simulink model "inverter_spwm_sixty_phases"  (R2024b)
settings: Solver=VariableStepAuto  StartTime=0.0  StopTime=0.1  RelTol=1e-3
libraries: spsMosfetLib x132, spsSeriesRLCBranchLib x65, spsCurrentMeasurementLib x64, spsVoltageMeasurementLib x64, spsTriangleGeneratorLib x20, spsDCVoltageSourceLib x4, spsGroundLib x2, spsThreePhaseSeriesRLCBranchLib x1, sps_lib x1
(part 2 of 2)

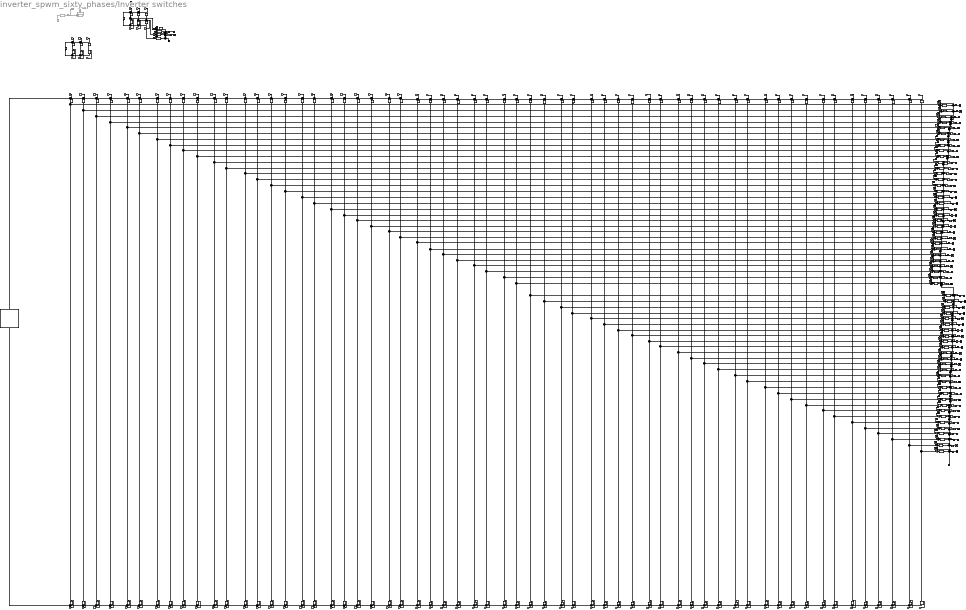
== system inverter_spwm_sixty_phases/Inverter switches ==
  Current Measurement : spsCurrentMeasurementLib/Current Measurement  Commented=on  PhasorSimulation=off  OutputType=Complex  PSBequivalent=0
  Current Measurement{1..47,49..52,55..66} (63 alike) : spsCurrentMeasurementLib/Current Measurement  PhasorSimulation=off  OutputType=Complex  PSBequivalent=0
  DC Voltage Source : spsDCVoltageSourceLib/DC Voltage Source  Amplitude=48  Measurements=None
  DC Voltage Source1 : spsDCVoltageSourceLib/DC Voltage Source  Commented=on  Amplitude=48  Measurements=None
  DC Voltage Source2 : spsDCVoltageSourceLib/DC Voltage Source  Amplitude=48  Measurements=None
  DC Voltage Source3 : spsDCVoltageSourceLib/DC Voltage Source  Amplitude=48  Measurements=None
  Ground : spsGroundLib/Ground  LConnTagsString=a
  Ground1 : spsGroundLib/Ground  LConnTagsString=a
  Mosfet{1..5,7..11,13..132} (130 alike) : spsMosfetLib/Mosfet  Ron=ron  Lon=0  Rd=rd  Vfd=fv  IC=0  Rs=0  Cs=0  Measurements=on
  Mosfet12 : spsMosfetLib/Mosfet  Ron=ron  Lon=0  Rd=rd  Vfd=fv  IC=0  Rs=0  Cs=0  Measurements=off
  Mosfet6 : spsMosfetLib/Mosfet  Ron=ron  Lon=0  Rd=rd  Vfd=fv  IC=0  Rs=0  Cs=0  Measurements=off
  Scope{,1,3..4,6..118,127..134} (125 alike) : Scope
  Scope2 : Scope  Commented=on
  Scope5 : Scope  Commented=on
  Series RLC Branch : spsSeriesRLCBranchLib/Series RLC Branch  Commented=on  LConnTagsString=__new0  RConnTagsString=__new0  BranchType=RC  Resistance=0.005  Inductance=0  SetiL0=off  InitialCurrent=0  Capacitance=0.02  Setx0=off  InitialVoltage=0  Measurements=None
  Series RLC Branch1 : spsSeriesRLCBranchLib/Series RLC Branch  Commented=on  LConnTagsString=__new0  RConnTagsString=__new0  BranchType=R  Resistance=0.0005  Inductance=1e-3  SetiL0=off  InitialCurrent=0  Capacitance=1e-6  Setx0=off  InitialVoltage=0  Measurements=None
  Series RLC Branch{2..50,54..57,59..68} (63 alike) : spsSeriesRLCBranchLib/Series RLC Branch  LConnTagsString=__new0  RConnTagsString=__new0  BranchType=RL  Resistance=1.0274  Inductance=0.0027  SetiL0=off  InitialCurrent=0  Capacitance=1e-6  Setx0=off  InitialVoltage=0  Measurements=None
  Three-Phase Series RLC Branch1 : spsThreePhaseSeriesRLCBranchLib/Three-Phase Series RLC Branch  LConnTagsString=A|B|C  RConnTagsString=A|B|C  BranchType=RL  Resistance=1.0274  Inductance=0.0027  Capacitance=1e-6  Measurements=Branch voltages
  Voltage Measurement : spsVoltageMeasurementLib/Voltage Measurement  Commented=on  PhasorSimulation=off  OutputType=Complex  PSBequivalent=0
  Voltage Measurement{1..47,50..53,56..67} (63 alike) : spsVoltageMeasurementLib/Voltage Measurement  PhasorSimulation=off  OutputType=Complex  PSBequivalent=0
  wires:
  [s6] -> Mosfet6/1
  [s1] -> Mosfet1/1
  [s3] -> Mosfet2/1
  [s5] -> Mosfet3/1
  [s2] -> Mosfet4/1
  [s4] -> Mosfet5/1
  Voltage Measurement/1 -> Scope5/1
  Current Measurement/1 -> Scope2/1
  Current Measurement1/1 -> Scope6/1
  Voltage Measurement2/1 -> Scope7/1
  Voltage Measurement3/1 -> Scope/1
  Current Measurement2/1 -> Scope1/1
  Current Measurement3/1 -> Scope3/1
  [s1] -> Mosfet7/1
  [s4] -> Mosfet11/1
  [s6] -> Mosfet12/1
  [s2] -> Mosfet10/1
  [s5] -> Mosfet9/1
  [s3] -> Mosfet8/1
  [s1] -> Mosfet13/1
  [s3] -> Mosfet14/1
  [s5] -> Mosfet17/1
  [s7] -> Mosfet19/1
  [s9] -> Mosfet21/1
  [s11] -> Mosfet23/1
  [s2] -> Mosfet15/1
  [s4] -> Mosfet16/1
  [s6] -> Mosfet18/1
  [s8] -> Mosfet20/1
  [s10] -> Mosfet22/1
  [s12] -> Mosfet24/1
  [s24] -> Mosfet36/1
  [s18] -> Mosfet30/1
  [s16] -> Mosfet28/1
  [s14] -> Mosfet27/1
  [s20] -> Mosfet32/1
  [s23] -> Mosfet35/1
  [s21] -> Mosfet33/1
  [s22] -> Mosfet34/1
  [s19] -> Mosfet31/1
  [s17] -> Mosfet29/1
  [s15] -> Mosfet26/1
  [s13] -> Mosfet25/1
  [s36] -> Mosfet48/1
  [s30] -> Mosfet42/1
  [s28] -> Mosfet40/1
  [s26] -> Mosfet39/1
  [s32] -> Mosfet44/1
  [s35] -> Mosfet47/1
  [s33] -> Mosfet45/1
  [s45] -> Mosfet57/1
  [s47] -> Mosfet59/1
  [s44] -> Mosfet56/1
  [s46] -> Mosfet58/1
  [s34] -> Mosfet46/1
  [s38] -> Mosfet51/1
  [s42] -> Mosfet54/1
  [s48] -> Mosfet60/1
  [s43] -> Mosfet55/1
  [s37] -> Mosfet49/1
  [s39] -> Mosfet50/1
  [s29] -> Mosfet41/1
  [s40] -> Mosfet52/1
  [s31] -> Mosfet43/1
  [s41] -> Mosfet53/1
  [s25] -> Mosfet37/1
  [s27] -> Mosfet38/1
  [s108] -> Mosfet72/1
  [s102] -> Mosfet66/1
  [s100] -> Mosfet64/1
  [s98] -> Mosfet63/1
  [s104] -> Mosfet68/1
  [s107] -> Mosfet71/1
  [s105] -> Mosfet69/1
  [s117] -> Mosfet81/1
  [s119] -> Mosfet83/1
  [s116] -> Mosfet80/1
  [s118] -> Mosfet82/1
  [s106] -> Mosfet70/1
  [s110] -> Mosfet75/1
  [s114] -> Mosfet78/1
  [s120] -> Mosfet84/1
  [s115] -> Mosfet79/1
  [s109] -> Mosfet73/1
  [s111] -> Mosfet74/1
  [s101] -> Mosfet65/1
  [s112] -> Mosfet76/1
  [s103] -> Mosfet67/1
  [s113] -> Mosfet77/1
  [s97] -> Mosfet61/1
  [s99] -> Mosfet62/1
  [s60] -> Mosfet96/1
  [s54] -> Mosfet90/1
  [s88] -> Mosfet124/1
  [s77] -> Mosfet113/1
  [s75] -> Mosfet110/1
  [s89] -> Mosfet125/1
  [s73] -> Mosfet109/1
  [s93] -> Mosfet129/1
  [s87] -> Mosfet122/1
  [s95] -> Mosfet131/1
  [s94] -> Mosfet130/1
  [s96] -> Mosfet132/1
  [s90] -> Mosfet126/1
  [s86] -> Mosfet123/1
  [s81] -> Mosfet117/1
  [s82] -> Mosfet118/1
  [s92] -> Mosfet128/1
  [s91] -> Mosfet127/1
  [s83] -> Mosfet119/1
  [s74] -> Mosfet111/1
  [s76] -> Mosfet112/1
  [s80] -> Mosfet116/1
  [s79] -> Mosfet115/1
  [s52] -> Mosfet88/1
  [s50] -> Mosfet87/1
  [s84] -> Mosfet120/1
  [s56] -> Mosfet92/1
  [s59] -> Mosfet95/1
  [s57] -> Mosfet93/1
  [s69] -> Mosfet105/1
  [s71] -> Mosfet107/1
  [s68] -> Mosfet104/1
  [s70] -> Mosfet106/1
  [s78] -> Mosfet114/1
  [s58] -> Mosfet94/1
  [s62] -> Mosfet99/1
  [s66] -> Mosfet102/1
  [s72] -> Mosfet108/1
  [s67] -> Mosfet103/1
  [s61] -> Mosfet97/1
  [s63] -> Mosfet98/1
  [s53] -> Mosfet89/1
  [s64] -> Mosfet100/1
  [s55] -> Mosfet91/1
  [s65] -> Mosfet101/1
  [s49] -> Mosfet85/1
  [s51] -> Mosfet86/1
  [s85] -> Mosfet121/1
  Current Measurement5/1 -> Scope10/1
  Voltage Measurement5/1 -> Scope9/1
  Voltage Measurement4/1 -> Scope8/1
  Current Measurement4/1 -> Scope4/1
  Current Measurement6/1 -> Scope12/1
  Voltage Measurement6/1 -> Scope13/1
  Voltage Measurement7/1 -> Scope14/1
  Current Measurement7/1 -> Scope11/1
  Current Measurement11/1 -> Scope16/1
  Voltage Measurement11/1 -> Scope19/1
  Voltage Measurement10/1 -> Scope18/1
  Current Measurement10/1 -> Scope17/1
  Current Measurement8/1 -> Scope20/1
  Voltage Measurement8/1 -> Scope21/1
  Voltage Measurement9/1 -> Scope22/1
  Current Measurement9/1 -> Scope15/1
  Current Measurement19/1 -> Scope28/1
  Voltage Measurement19/1 -> Scope35/1
  Voltage Measurement18/1 -> Scope34/1
  Current Measurement18/1 -> Scope33/1
  Current Measurement12/1 -> Scope30/1
  Voltage Measurement12/1 -> Scope31/1
  Voltage Measurement13/1 -> Scope32/1
  Current Measurement13/1 -> Scope29/1
  Current Measurement17/1 -> Scope24/1
  Voltage Measurement17/1 -> Scope27/1
  Voltage Measurement16/1 -> Scope26/1
  Current Measurement16/1 -> Scope25/1
  Current Measurement14/1 -> Scope36/1
  Voltage Measurement14/1 -> Scope37/1
  Voltage Measurement15/1 -> Scope38/1
  Current Measurement15/1 -> Scope23/1
  Current Measurement25/1 -> Scope52/1
  Voltage Measurement25/1 -> Scope67/1
  Voltage Measurement24/1 -> Scope66/1
  Current Measurement24/1 -> Scope65/1
  Current Measurement26/1 -> Scope54/1
  Voltage Measurement26/1 -> Scope55/1
  Voltage Measurement27/1 -> Scope56/1
  Current Measurement27/1 -> Scope53/1
  Current Measurement23/1 -> Scope58/1
  Voltage Measurement23/1 -> Scope61/1
  Voltage Measurement22/1 -> Scope60/1
  Current Measurement22/1 -> Scope59/1
  Current Measurement28/1 -> Scope62/1
  Voltage Measurement28/1 -> Scope63/1
  Voltage Measurement29/1 -> Scope64/1
  Current Measurement29/1 -> Scope57/1
  Current Measurement35/1 -> Scope44/1
  Voltage Measurement35/1 -> Scope51/1
  Voltage Measurement34/1 -> Scope50/1
  Current Measurement34/1 -> Scope49/1
  Current Measurement20/1 -> Scope46/1
  Voltage Measurement20/1 -> Scope47/1
  Voltage Measurement21/1 -> Scope48/1
  Current Measurement21/1 -> Scope45/1
  Current Measurement33/1 -> Scope40/1
  Voltage Measurement33/1 -> Scope43/1
  Voltage Measurement32/1 -> Scope42/1
  Current Measurement32/1 -> Scope41/1
  Current Measurement30/1 -> Scope68/1
  Voltage Measurement30/1 -> Scope69/1
  Voltage Measurement31/1 -> Scope70/1
  Current Measurement31/1 -> Scope39/1
  Current Measurement56/1 -> Scope100/1
  Voltage Measurement57/1 -> Scope132/1
  Voltage Measurement56/1 -> Scope131/1
  Current Measurement55/1 -> Scope130/1
  Current Measurement57/1 -> Scope103/1
  Voltage Measurement58/1 -> Scope104/1
  Voltage Measurement59/1 -> Scope105/1
  Current Measurement58/1 -> Scope102/1
  Current Measurement47/1 -> Scope107/1
  Voltage Measurement47/1 -> Scope110/1
  Voltage Measurement46/1 -> Scope109/1
  Current Measurement46/1 -> Scope108/1
  Current Measurement59/1 -> Scope111/1
  Voltage Measurement60/1 -> Scope112/1
  Voltage Measurement61/1 -> Scope113/1
  Current Measurement60/1 -> Scope106/1
  Current Measurement52/1 -> Scope115/1
  Voltage Measurement53/1 -> Scope118/1
  Voltage Measurement52/1 -> Scope117/1
  Current Measurement51/1 -> Scope116/1
  Current Measurement49/1 -> Scope127/1
  Voltage Measurement50/1 -> Scope128/1
  Voltage Measurement51/1 -> Scope129/1
  Current Measurement50/1 -> Scope114/1
  Current Measurement41/1 -> Scope84/1
  Voltage Measurement41/1 -> Scope99/1
  Voltage Measurement40/1 -> Scope98/1
  Current Measurement40/1 -> Scope97/1
  Current Measurement42/1 -> Scope86/1
  Voltage Measurement42/1 -> Scope87/1
  Voltage Measurement43/1 -> Scope88/1
  Current Measurement43/1 -> Scope85/1
  Current Measurement39/1 -> Scope90/1
  Voltage Measurement39/1 -> Scope93/1
  Voltage Measurement38/1 -> Scope92/1
  Current Measurement38/1 -> Scope91/1
  Current Measurement44/1 -> Scope94/1
  Voltage Measurement44/1 -> Scope95/1
  Voltage Measurement45/1 -> Scope96/1
  Current Measurement45/1 -> Scope89/1
  Current Measurement66/1 -> Scope76/1
  Voltage Measurement67/1 -> Scope83/1
  Voltage Measurement66/1 -> Scope82/1
  Current Measurement65/1 -> Scope81/1
  Current Measurement36/1 -> Scope78/1
  Voltage Measurement36/1 -> Scope79/1
  Voltage Measurement37/1 -> Scope80/1
  Current Measurement37/1 -> Scope77/1
  Current Measurement64/1 -> Scope72/1
  Voltage Measurement65/1 -> Scope75/1
  Voltage Measurement64/1 -> Scope74/1
  Current Measurement63/1 -> Scope73/1
  Current Measurement61/1 -> Scope101/1
  Voltage Measurement62/1 -> Scope133/1
  Voltage Measurement63/1 -> Scope134/1
  Current Measurement62/1 -> Scope71/1
  connections:
  Mosfet2/LConn1 -- DC Voltage Source/RConn1 -- Mosfet1/LConn1 -- Mosfet3/LConn1
  Mosfet3/RConn1 -- Current Measurement3/LConn1 -- Mosfet6/LConn1
  Mosfet2/RConn1 -- Current Measurement2/LConn1 -- Mosfet5/LConn1
  Mosfet1/RConn1 -- Current Measurement1/LConn1 -- Mosfet4/LConn1
  Mosfet5/RConn1 -- Mosfet4/RConn1 -- DC Voltage Source/LConn1 -- Mosfet6/RConn1
  Current Measurement/RConn1 -- Voltage Measurement/LConn1 -- Series RLC Branch/LConn1
  Voltage Measurement/LConn2 -- Series RLC Branch/RConn1
  Series RLC Branch1/RConn1 -- Current Measurement/LConn1
  DC Voltage Source1/RConn1 -- Series RLC Branch1/LConn1
  Current Measurement1/RConn1 -- Voltage Measurement2/LConn1 -- Series RLC Branch2/LConn1
  Voltage Measurement2/LConn2 -- Series RLC Branch4/RConn1 -- Ground/LConn1 -- Voltage Measurement3/LConn2 -- Series RLC Branch3/RConn1 -- Series RLC Branch2/RConn1
  Series RLC Branch3/LConn1 -- Voltage Measurement3/LConn1 -- Current Measurement2/RConn1
  Series RLC Branch4/LConn1 -- Current Measurement3/RConn1
  Mosfet12/LConn1 -- Mosfet9/RConn1
  DC Voltage Source2/LConn1 -- Mosfet11/RConn1 -- Mosfet12/RConn1 -- Mosfet10/RConn1
  Mosfet9/LConn1 -- Mosfet8/LConn1 -- DC Voltage Source2/RConn1 -- Mosfet7/LConn1
  Mosfet11/LConn1 -- Mosfet8/RConn1
  Mosfet7/RConn1 -- Mosfet10/LConn1
  Mosfet15/LConn1 -- Current Measurement5/LConn1 -- Mosfet13/RConn1
  Mosfet16/LConn1 -- Mosfet14/RConn1 -- Current Measurement4/LConn1
  Mosfet18/LConn1 -- Mosfet17/RConn1 -- Current Measurement7/LConn1
  Current Measurement55/LConn1 -- Mosfet64/LConn1 -- Mosfet62/RConn1
  Current Measurement60/LConn1 -- Mosfet70/LConn1 -- Mosfet69/RConn1
  Current Measurement38/LConn1 -- Mosfet132/LConn1 -- Mosfet131/RConn1
  Mosfet80/LConn1 -- Current Measurement49/LConn1 -- Mosfet79/RConn1
  Mosfet82/LConn1 -- Mosfet81/RConn1 -- Current Measurement52/LConn1
  Mosfet84/LConn1 -- Mosfet83/RConn1 -- Current Measurement51/LConn1
  Current Measurement57/LConn1 -- Mosfet68/LConn1 -- Mosfet67/RConn1
  Current Measurement46/LConn1 -- Mosfet76/LConn1 -- Mosfet74/RConn1
  Mosfet81/LConn1 -- Mosfet83/LConn1 -- Mosfet79/LConn1 -- Mosfet77/LConn1 -- Mosfet73/LConn1 -- Mosfet61/LConn1 -- Mosfet129/LConn1 -- Mosfet127/LConn1 -- Mosfet125/LConn1 -- Mosfet122/LConn1 -- Mosfet121/LConn1 -- Mosfet119/LConn1 -- Mosfet117/LConn1 -- Mosfet97/LConn1 -- Mosfet85/LConn1 -- Mosfet49/LConn1 -- Mosfet25/LConn1 -- DC Voltage Source3/RConn1 -- Mosfet13/LConn1 -- Mosfet14/LConn1 -- Mosfet17/LConn1 -- Mosfet19/LConn1 -- Mosfet21/LConn1 -- Mosfet23/LConn1 -- Mosfet26/LConn1 -- Mosfet29/LConn1 -- Mosfet31/LConn1 -- Mosfet33/LConn1 -- Mosfet35/LConn1 -- Mosfet37/LConn1 -- Mosfet38/LConn1 -- Mosfet41/LConn1 -- Mosfet43/LConn1 -- Mosfet45/LConn1 -- Mosfet47/LConn1 -- Mosfet50/LConn1 -- Mosfet53/LConn1 -- Mosfet55/LConn1 -- Mosfet57/LConn1 -- Mosfet59/LConn1 -- Mosfet86/LConn1 -- Mosfet89/LConn1 -- Mosfet91/LConn1 -- Mosfet93/LConn1 -- Mosfet95/LConn1 -- Mosfet98/LConn1 -- Mosfet101/LConn1 -- Mosfet103/LConn1 -- Mosfet105/LConn1 -- Mosfet107/LConn1 -- Mosfet109/LConn1 -- Mosfet110/LConn1 -- Mosfet113/LConn1 -- Mosfet115/LConn1 -- Mosfet131/LConn1 -- Mosfet62/LConn1 -- Mosfet65/LConn1 -- Mosfet67/LConn1 -- Mosfet69/LConn1 -- Mosfet71/LConn1 -- Mosfet74/LConn1
  Mosfet66/RConn1 -- Mosfet64/RConn1 -- Mosfet63/RConn1 -- Mosfet124/RConn1 -- Mosfet112/RConn1 -- Mosfet100/RConn1 -- Mosfet88/RConn1 -- Mosfet52/RConn1 -- Mosfet40/RConn1 -- Mosfet28/RConn1 -- Mosfet16/RConn1 -- Mosfet15/RConn1 -- DC Voltage Source3/LConn1 -- Mosfet18/RConn1 -- Mosfet20/RConn1 -- Mosfet22/RConn1 -- Mosfet24/RConn1 -- Mosfet27/RConn1 -- Mosfet30/RConn1 -- Mosfet32/RConn1 -- Mosfet34/RConn1 -- Mosfet36/RConn1 -- Mosfet39/RConn1 -- Mosfet42/RConn1 -- Mosfet44/RConn1 -- Mosfet46/RConn1 -- Mosfet48/RConn1 -- Mosfet51/RConn1 -- Mosfet54/RConn1 -- Mosfet56/RConn1 -- Mosfet58/RConn1 -- Mosfet60/RConn1 -- Mosfet87/RConn1 -- Mosfet90/RConn1 -- Mosfet92/RConn1 -- Mosfet94/RConn1 -- Mosfet96/RConn1 -- Mosfet99/RConn1 -- Mosfet102/RConn1 -- Mosfet104/RConn1 -- Mosfet106/RConn1 -- Mosfet108/RConn1 -- Mosfet111/RConn1 -- Mosfet114/RConn1 -- Mosfet116/RConn1 -- Mosfet118/RConn1 -- Mosfet120/RConn1 -- Mosfet123/RConn1 -- Mosfet126/RConn1 -- Mosfet128/RConn1 -- Mosfet130/RConn1 -- Mosfet132/RConn1 -- Mosfet76/RConn1 -- Mosfet84/RConn1 -- Mosfet82/RConn1 -- Mosfet80/RConn1 -- Mosfet78/RConn1 -- Mosfet75/RConn1 -- Mosfet72/RConn1 -- Mosfet70/RConn1 -- Mosfet68/RConn1
  Current Measurement44/LConn1 -- Mosfet128/LConn1 -- Mosfet127/RConn1
  Current Measurement45/LConn1 -- Mosfet126/LConn1 -- Mosfet125/RConn1
  Current Measurement36/LConn1 -- Mosfet116/LConn1 -- Mosfet115/RConn1
  Current Measurement39/LConn1 -- Mosfet130/LConn1 -- Mosfet129/RConn1
  Current Measurement43/LConn1 -- Mosfet123/LConn1 -- Mosfet121/RConn1
  Current Measurement41/LConn1 -- Mosfet118/LConn1 -- Mosfet117/RConn1
  Voltage Measurement5/LConn1 -- Series RLC Branch6/LConn1 -- Current Measurement5/RConn1
  Series RLC Branch35/RConn1 -- Voltage Measurement35/LConn2 -- Series RLC Branch21/RConn1 -- Series RLC Branch36/RConn1 -- Voltage Measurement24/LConn2 -- Series RLC Branch27/RConn1 -- Voltage Measurement22/LConn2 -- Series RLC Branch25/RConn1 -- Voltage Measurement62/LConn2 -- Series RLC Branch64/RConn1 -- Voltage Measurement64/LConn2 -- Series RLC Branch66/RConn1 -- Voltage Measurement67/LConn2 -- Series RLC Branch37/RConn1 -- Voltage Measurement43/LConn2 -- Series RLC Branch46/RConn1 -- Voltage Measurement45/LConn2 -- Series RLC Branch40/RConn1 -- Voltage Measurement44/LConn2 -- Series RLC Branch47/RConn1 -- Voltage Measurement56/LConn2 -- Series RLC Branch59/RConn1 -- Voltage Measurement59/LConn2 -- Series RLC Branch62/RConn1 -- Voltage Measurement58/LConn2 -- Series RLC Branch61/RConn1 -- Voltage Measurement61/LConn2 -- Series RLC Branch48/RConn1 -- Voltage Measurement60/LConn2 -- Series RLC Branch63/RConn1 -- Ground1/LConn1 -- Voltage Measurement52/LConn2 -- Series RLC Branch56/RConn1 -- Voltage Measurement53/LConn2 -- Series RLC Branch57/RConn1 -- Voltage Measurement50/LConn2 -- Series RLC Branch54/RConn1 -- Voltage Measurement51/LConn2 -- Series RLC Branch55/RConn1 -- Voltage Measurement46/LConn2 -- Series RLC Branch49/RConn1 -- Voltage Measurement47/LConn2 -- Series RLC Branch50/RConn1 -- Voltage Measurement57/LConn2 -- Series RLC Branch60/RConn1 -- Voltage Measurement38/LConn2 -- Series RLC Branch41/RConn1 -- Voltage Measurement39/LConn2 -- Series RLC Branch42/RConn1 -- Voltage Measurement42/LConn2 -- Series RLC Branch45/RConn1 -- Voltage Measurement40/LConn2 -- Series RLC Branch43/RConn1 -- Voltage Measurement41/LConn2 -- Series RLC Branch44/RConn1 -- Voltage Measurement36/LConn2 -- Series RLC Branch38/RConn1 -- Voltage Measurement37/LConn2 -- Series RLC Branch39/RConn1 -- Voltage Measurement66/LConn2 -- Series RLC Branch68/RConn1 -- Voltage Measurement65/LConn2 -- Series RLC Branch67/RConn1 -- Voltage Measurement63/LConn2 -- Series RLC Branch65/RConn1 -- Voltage Measurement23/LConn2 -- Series RLC Branch26/RConn1 -- Voltage Measurement28/LConn2 -- Series RLC Branch31/RConn1 -- Voltage Measurement29/LConn2 -- Series RLC Branch24/RConn1 -- Voltage Measurement26/LConn2 -- Series RLC Branch29/RConn1 -- Voltage Measurement27/LConn2 -- Series RLC Branch30/RConn1 -- Voltage Measurement25/LConn2 -- Series RLC Branch28/RConn1 -- Voltage Measurement20/LConn2 -- Series RLC Branch22/RConn1 -- Series RLC Branch23/RConn1 -- Voltage Measurement21/LConn2 -- Voltage Measurement34/LConn2 -- Voltage Measurement32/LConn2 -- Series RLC Branch34/RConn1 -- Voltage Measurement5/LConn2 -- Series RLC Branch6/RConn1 -- Voltage Measurement4/LConn2 -- Series RLC Branch5/RConn1 -- Voltage Measurement7/LConn2 -- Series RLC Branch8/RConn1 -- Voltage Measurement6/LConn2 -- Series RLC Branch7/RConn1 -- Series RLC Branch10/RConn1 -- Voltage Measurement9/LConn2 -- Voltage Measurement8/LConn2 -- Series RLC Branch9/RConn1 -- Voltage Measurement11/LConn2 -- Series RLC Branch12/RConn1 -- Voltage Measurement10/LConn2 -- Series RLC Branch11/RConn1 -- Voltage Measurement15/LConn2 -- Series RLC Branch17/RConn1 -- Voltage Measurement14/LConn2 -- Series RLC Branch16/RConn1 -- Voltage Measurement17/LConn2 -- Series RLC Branch19/RConn1 -- Voltage Measurement16/LConn2 -- Series RLC Branch18/RConn1 -- Voltage Measurement19/LConn2 -- Series RLC Branch13/RConn1 -- Voltage Measurement18/LConn2 -- Series RLC Branch20/RConn1 -- Voltage Measurement13/LConn2 -- Series RLC Branch15/RConn1 -- Series RLC Branch14/RConn1 -- Voltage Measurement12/LConn2 -- Voltage Measurement31/LConn2 -- Series RLC Branch33/RConn1 -- Voltage Measurement30/LConn2 -- Series RLC Branch32/RConn1 -- Voltage Measurement33/LConn2
  Voltage Measurement4/LConn1 -- Series RLC Branch5/LConn1 -- Current Measurement4/RConn1
  Series RLC Branch8/LConn1 -- Voltage Measurement7/LConn1 -- Current Measurement7/RConn1
  Series RLC Branch7/LConn1 -- Voltage Measurement6/LConn1 -- Current Measurement6/RConn1
  Series RLC Branch10/LConn1 -- Voltage Measurement9/LConn1 -- Current Measurement9/RConn1
  Series RLC Branch9/LConn1 -- Voltage Measurement8/LConn1 -- Current Measurement8/RConn1
  Voltage Measurement11/LConn1 -- Series RLC Branch12/LConn1 -- Current Measurement11/RConn1
  Voltage Measurement10/LConn1 -- Series RLC Branch11/LConn1 -- Current Measurement10/RConn1
  Series RLC Branch17/LConn1 -- Voltage Measurement15/LConn1 -- Current Measurement15/RConn1
  Series RLC Branch16/LConn1 -- Voltage Measurement14/LConn1 -- Current Measurement14/RConn1
  Voltage Measurement17/LConn1 -- Series RLC Branch19/LConn1 -- Current Measurement17/RConn1
  Voltage Measurement16/LConn1 -- Series RLC Branch18/LConn1 -- Current Measurement16/RConn1
  Voltage Measurement19/LConn1 -- Series RLC Branch13/LConn1 -- Current Measurement19/RConn1
  Voltage Measurement18/LConn1 -- Series RLC Branch20/LConn1 -- Current Measurement18/RConn1
  Series RLC Branch15/LConn1 -- Voltage Measurement13/LConn1 -- Current Measurement13/RConn1
  Series RLC Branch14/LConn1 -- Voltage Measurement12/LConn1 -- Current Measurement12/RConn1
  Series RLC Branch33/LConn1 -- Voltage Measurement31/LConn1 -- Current Measurement31/RConn1
  Series RLC Branch32/LConn1 -- Voltage Measurement30/LConn1 -- Current Measurement30/RConn1
  Voltage Measurement33/LConn1 -- Series RLC Branch35/LConn1 -- Current Measurement33/RConn1
  Voltage Measurement32/LConn1 -- Series RLC Branch34/LConn1 -- Current Measurement32/RConn1
  Voltage Measurement35/LConn1 -- Series RLC Branch21/LConn1 -- Current Measurement35/RConn1
  Voltage Measurement34/LConn1 -- Series RLC Branch36/LConn1 -- Current Measurement34/RConn1
  Series RLC Branch23/LConn1 -- Voltage Measurement21/LConn1 -- Current Measurement21/RConn1
  Series RLC Branch22/LConn1 -- Voltage Measurement20/LConn1 -- Current Measurement20/RConn1
  Voltage Measurement25/LConn1 -- Series RLC Branch28/LConn1 -- Current Measurement25/RConn1
  Voltage Measurement24/LConn1 -- Series RLC Branch27/LConn1 -- Current Measurement24/RConn1
  Series RLC Branch30/LConn1 -- Voltage Measurement27/LConn1 -- Current Measurement27/RConn1
  Series RLC Branch29/LConn1 -- Voltage Measurement26/LConn1 -- Current Measurement26/RConn1
  Series RLC Branch24/LConn1 -- Voltage Measurement29/LConn1 -- Current Measurement29/RConn1
  Series RLC Branch31/LConn1 -- Voltage Measurement28/LConn1 -- Current Measurement28/RConn1
  Voltage Measurement23/LConn1 -- Series RLC Branch26/LConn1 -- Current Measurement23/RConn1
  Voltage Measurement22/LConn1 -- Series RLC Branch25/LConn1 -- Current Measurement22/RConn1
  Series RLC Branch65/LConn1 -- Voltage Measurement63/LConn1 -- Current Measurement62/RConn1
  Series RLC Branch64/LConn1 -- Voltage Measurement62/LConn1 -- Current Measurement61/RConn1
  Voltage Measurement65/LConn1 -- Series RLC Branch67/LConn1 -- Current Measurement64/RConn1
  Voltage Measurement64/LConn1 -- Series RLC Branch66/LConn1 -- Current Measurement63/RConn1
  Voltage Measurement67/LConn1 -- Series RLC Branch37/LConn1 -- Current Measurement66/RConn1
  Voltage Measurement66/LConn1 -- Series RLC Branch68/LConn1 -- Current Measurement65/RConn1
  Series RLC Branch39/LConn1 -- Voltage Measurement37/LConn1 -- Current Measurement37/RConn1
  Series RLC Branch38/LConn1 -- Voltage Measurement36/LConn1 -- Current Measurement36/RConn1
  Voltage Measurement41/LConn1 -- Series RLC Branch44/LConn1 -- Current Measurement41/RConn1
  Voltage Measurement40/LConn1 -- Series RLC Branch43/LConn1 -- Current Measurement40/RConn1
  Series RLC Branch46/LConn1 -- Voltage Measurement43/LConn1 -- Current Measurement43/RConn1
  Series RLC Branch45/LConn1 -- Voltage Measurement42/LConn1 -- Current Measurement42/RConn1
  Series RLC Branch40/LConn1 -- Voltage Measurement45/LConn1 -- Current Measurement45/RConn1
  Series RLC Branch47/LConn1 -- Voltage Measurement44/LConn1 -- Current Measurement44/RConn1
  Voltage Measurement39/LConn1 -- Series RLC Branch42/LConn1 -- Current Measurement39/RConn1
  Voltage Measurement38/LConn1 -- Series RLC Branch41/LConn1 -- Current Measurement38/RConn1
  Voltage Measurement57/LConn1 -- Series RLC Branch60/LConn1 -- Current Measurement56/RConn1
  Voltage Measurement56/LConn1 -- Series RLC Branch59/LConn1 -- Current Measurement55/RConn1
  Series RLC Branch62/LConn1 -- Voltage Measurement59/LConn1 -- Current Measurement58/RConn1
  Series RLC Branch61/LConn1 -- Voltage Measurement58/LConn1 -- Current Measurement57/RConn1
  Series RLC Branch48/LConn1 -- Voltage Measurement61/LConn1 -- Current Measurement60/RConn1
  Series RLC Branch63/LConn1 -- Voltage Measurement60/LConn1 -- Current Measurement59/RConn1
  Voltage Measurement47/LConn1 -- Series RLC Branch50/LConn1 -- Current Measurement47/RConn1
  Voltage Measurement46/LConn1 -- Series RLC Branch49/LConn1 -- Current Measurement46/RConn1
  Series RLC Branch55/LConn1 -- Voltage Measurement51/LConn1 -- Current Measurement50/RConn1
  Series RLC Branch54/LConn1 -- Voltage Measurement50/LConn1 -- Current Measurement49/RConn1
  Voltage Measurement53/LConn1 -- Series RLC Branch57/LConn1 -- Current Measurement52/RConn1
  Voltage Measurement52/LConn1 -- Series RLC Branch56/LConn1 -- Current Measurement51/RConn1
  Current Measurement9/LConn1 -- Mosfet21/RConn1 -- Mosfet22/LConn1
  Mosfet19/RConn1 -- Mosfet20/LConn1 -- Current Measurement6/LConn1
  Mosfet27/LConn1 -- Current Measurement11/LConn1 -- Mosfet25/RConn1
  Mosfet24/LConn1 -- Current Measurement8/LConn1 -- Mosfet23/RConn1
  Mosfet28/LConn1 -- Current Measurement10/LConn1 -- Mosfet26/RConn1
  Mosfet30/LConn1 -- Mosfet29/RConn1 -- Current Measurement15/LConn1
  Current Measurement14/LConn1 -- Mosfet31/RConn1 -- Mosfet32/LConn1
  Current Measurement17/LConn1 -- Mosfet33/RConn1 -- Mosfet34/LConn1
  Current Measurement16/LConn1 -- Mosfet35/RConn1 -- Mosfet36/LConn1
  Mosfet39/LConn1 -- Current Measurement19/LConn1 -- Mosfet37/RConn1
  Mosfet42/LConn1 -- Current Measurement13/LConn1 -- Mosfet41/RConn1
  Mosfet40/LConn1 -- Mosfet38/RConn1 -- Current Measurement18/LConn1
  Current Measurement30/LConn1 -- Mosfet47/RConn1 -- Mosfet48/LConn1
  Current Measurement12/LConn1 -- Mosfet43/RConn1 -- Mosfet44/LConn1
  Mosfet46/LConn1 -- Current Measurement31/LConn1 -- Mosfet45/RConn1
  Current Measurement32/LConn1 -- Mosfet50/RConn1 -- Mosfet52/LConn1
  Mosfet51/LConn1 -- Current Measurement33/LConn1 -- Mosfet49/RConn1
  Current Measurement35/LConn1 -- Mosfet53/RConn1 -- Mosfet54/LConn1
  Current Measurement21/LConn1 -- Mosfet58/LConn1 -- Mosfet57/RConn1
  Mosfet56/LConn1 -- Current Measurement34/LConn1 -- Mosfet55/RConn1
  Current Measurement20/LConn1 -- Mosfet60/LConn1 -- Mosfet59/RConn1
  Current Measurement24/LConn1 -- Mosfet86/RConn1 -- Mosfet88/LConn1
  Current Measurement25/LConn1 -- Mosfet85/RConn1 -- Mosfet87/LConn1
  Mosfet89/RConn1 -- Mosfet90/LConn1 -- Current Measurement27/LConn1
  Current Measurement29/LConn1 -- Mosfet93/RConn1 -- Mosfet94/LConn1
  Current Measurement26/LConn1 -- Mosfet92/LConn1 -- Mosfet91/RConn1
  Current Measurement28/LConn1 -- Mosfet95/RConn1 -- Mosfet96/LConn1
  Mosfet97/RConn1 -- Mosfet99/LConn1 -- Current Measurement23/LConn1
  Current Measurement22/LConn1 -- Mosfet98/RConn1 -- Mosfet100/LConn1
  Current Measurement61/LConn1 -- Mosfet103/RConn1 -- Mosfet104/LConn1
  Current Measurement62/LConn1 -- Mosfet101/RConn1 -- Mosfet102/LConn1
  Current Measurement64/LConn1 -- Mosfet105/RConn1 -- Mosfet106/LConn1
  Current Measurement66/LConn1 -- Mosfet109/RConn1 -- Mosfet111/LConn1
  Current Measurement63/LConn1 -- Mosfet107/RConn1 -- Mosfet108/LConn1
  Mosfet110/RConn1 -- Mosfet112/LConn1 -- Current Measurement65/LConn1
  Current Measurement37/LConn1 -- Mosfet114/LConn1 -- Mosfet113/RConn1
  Current Measurement40/LConn1 -- Mosfet120/LConn1 -- Mosfet119/RConn1
  Current Measurement42/LConn1 -- Mosfet124/LConn1 -- Mosfet122/RConn1
  Current Measurement56/LConn1 -- Mosfet63/LConn1 -- Mosfet61/RConn1
  Current Measurement58/LConn1 -- Mosfet66/LConn1 -- Mosfet65/RConn1
  Mosfet72/LConn1 -- Current Measurement59/LConn1 -- Mosfet71/RConn1
  Current Measurement47/LConn1 -- Mosfet75/LConn1 -- Mosfet73/RConn1
  Mosfet78/LConn1 -- Current Measurement50/LConn1 -- Mosfet77/RConn1
